simulink subsystem "ss_controller_robtracking"  (R2024b)
settings: Solver=VariableStepAuto  StartTime=0.0  StopTime=10.0  RelTol=1e-3
values from neighbouring files (symbols this model uses):
  A_q = Hss.A    [A_final_results.m]
  B_q = [zeros(2,1), Hss.B, zeros(2)]    [A_final_results.m]
  K_fb = lqr(Ae, Be, Qe, Re)    [A_final_results.m]
  Nu = Sol(7,:)    [A_final_results.m]
  Nx = Sol(1:6, :)    [A_final_results.m]
undefined symbols (not defined in the file or in its folder): rpm2rads
settings Model: Creator=Utente  LastModifiedBy=Buton

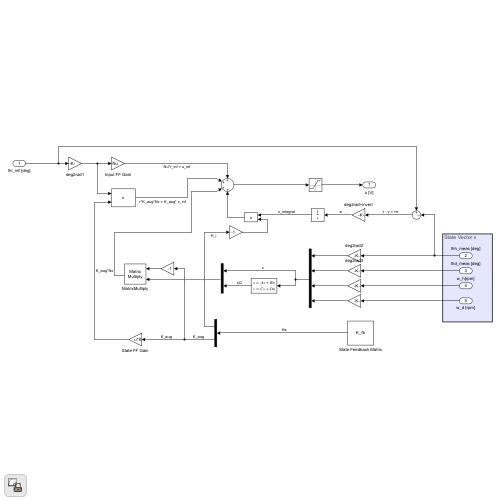
[thumbnail: Simulink's stored preview of the top-level diagram]
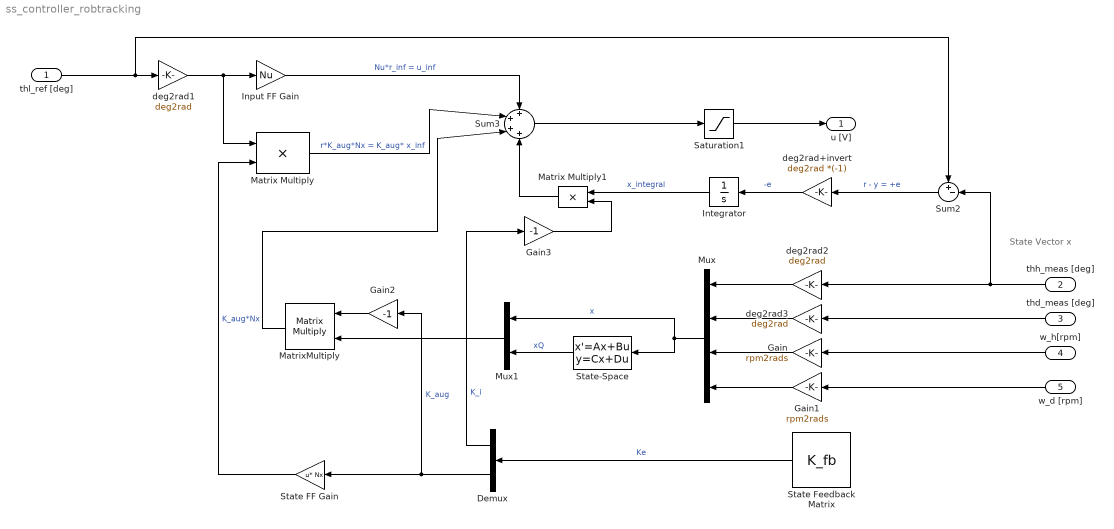
== system ss_controller_robtracking ==
  note: State Vector x
  thl_ref [deg] : Inport
  thh_meas [deg] : Inport  Port=2
  thd_meas [deg] : Inport  Port=3
  w_h[rpm] : Inport  Port=4
  w_d [rpm] : Inport  Port=5
  Demux : Demux  Outputs=2
  Gain : Gain  Gain=rpm2rads
  Gain1 : Gain  Gain=rpm2rads
  Gain2 : Gain  Gain=-1
  Gain3 : Gain  Gain=-1
  Input FF Gain : Gain  Gain=Nu
  Integrator : Integrator
  Matrix Multiply : Product
  Matrix Multiply1 : Product
  MatrixMultiply : Product  Multiplication=Matrix(*)
  Mux : Mux
  Mux1 : Mux  Inputs=2
  Saturation1 : Saturate  UpperLimit=12  LowerLimit=-12
  State FF Gain : Gain  Gain=Nx  Multiplication=Matrix(u*K)
  State Feedback Matrix : Constant  Value=K_fb
  State-Space : StateSpace  A=A_q  B=B_q  C=eye(2,2)  D=zeros(2,4)  InitialCondition=0
  Sum2 : Sum  Inputs=+-|
  Sum3 : Sum  Inputs=++++
  deg2rad+invert : Gain  Gain=deg2rad *(-1)
  deg2rad1 : Gain  Gain=deg2rad
  deg2rad2 : Gain  Gain=deg2rad
  deg2rad3 : Gain  Gain=deg2rad
  u [V] : Outport
  wires:
  deg2rad1/1 -> Input FF Gain/1, Matrix Multiply/1
  Saturation1/1 -> u [V]/1
  Integrator/1 -> Matrix Multiply1/1  "x_integral"
  State Feedback Matrix/1 -> Demux/1  "Ke"
  Matrix Multiply1/1 -> Sum3/4
  deg2rad+invert/1 -> Integrator/1  "-e"
  Sum3/1 -> Saturation1/1
  Demux/1 -> Gain3/1  "K_i"
  Input FF Gain/1 -> Sum3/1  "Nu*r_inf = u_inf"
  thl_ref [deg]/1 -> deg2rad1/1, Sum2/1
  State FF Gain/1 -> Matrix Multiply/2  "K_aug*Nx"
  Matrix Multiply/1 -> Sum3/2  "r*K_aug*Nx = K_aug* x_inf"
  Demux/2 -> State FF Gain/1, Gain2/1  "K_aug"
  MatrixMultiply/1 -> Sum3/3
  Gain3/1 -> Matrix Multiply1/2
  Sum2/1 -> deg2rad+invert/1  "r - y = +e"
  thd_meas [deg]/1 -> deg2rad3/1
  thh_meas [deg]/1 -> deg2rad2/1, Sum2/2
  Gain1/1 -> Mux/4
  w_d [rpm]/1 -> Gain1/1
  w_h[rpm]/1 -> Gain/1
  deg2rad2/1 -> Mux/1
  Gain/1 -> Mux/3
  deg2rad3/1 -> Mux/2
  Gain2/1 -> MatrixMultiply/1
  Mux/1 -> State-Space/1, Mux1/1  "x"
  State-Space/1 -> Mux1/2  "xQ"
  Mux1/1 -> MatrixMultiply/2
